simulink model "mux"  (R2023b)
settings: Solver=VariableStepAuto  StartTime=0.0  StopTime=1  RelTol=1e-3
settings Model: Creator=1234  LastModifiedBy=1234

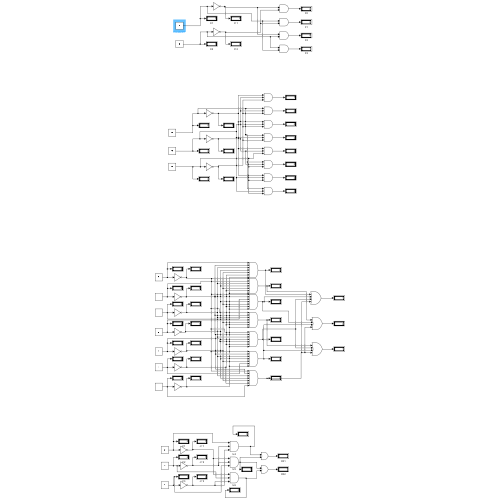
[thumbnail: Simulink's stored preview of the top-level diagram]
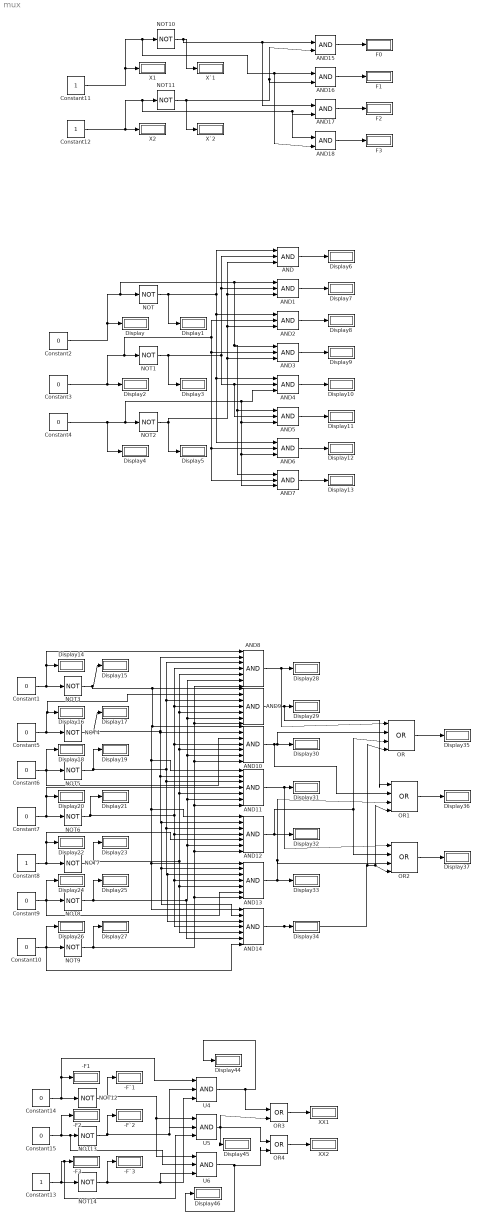
== system mux ==
  -F1 : Display
  -F2 : Display
  -F3 : Display
  -F`1 : Display
  -F`2 : Display
  -F`3 : Display
  AND{,1..7} (8 alike) : Logic  Inputs=3  IconShape=distinctive  AllPortsSameDT=off  OutDataTypeStr=boolean
  AND{8..14} (7 alike) : Logic  Inputs=7  IconShape=distinctive  AllPortsSameDT=off  OutDataTypeStr=boolean
  AND{15..18} (4 alike) : Logic  IconShape=distinctive  AllPortsSameDT=off  OutDataTypeStr=boolean
  Constant{1..7,9..10,14..15} (11 alike) : Constant  Value=0
  Constant{8,11..13} (4 alike) : Constant
  Display{,1..37,44..46} (41 alike) : Display
  F{0..3} (4 alike) : Display
  NOT{,1..14} (15 alike) : Logic  Operator=NOT  IconShape=distinctive  AllPortsSameDT=off  OutDataTypeStr=boolean
  OR : Logic  Operator=OR  Inputs=4  IconShape=distinctive  AllPortsSameDT=off  OutDataTypeStr=boolean
  OR1 : Logic  Operator=OR  Inputs=4  IconShape=distinctive  AllPortsSameDT=off  OutDataTypeStr=boolean
  OR2 : Logic  Operator=OR  Inputs=4  IconShape=distinctive  AllPortsSameDT=off  OutDataTypeStr=boolean
  OR3 : Logic  Operator=OR  IconShape=distinctive  AllPortsSameDT=off  OutDataTypeStr=boolean
  OR4 : Logic  Operator=OR  IconShape=distinctive  AllPortsSameDT=off  OutDataTypeStr=boolean
  U4 : Logic  Inputs=3  IconShape=distinctive  AllPortsSameDT=off  OutDataTypeStr=boolean
  U5 : Logic  Inputs=3  IconShape=distinctive  AllPortsSameDT=off  OutDataTypeStr=boolean
  U6 : Logic  Inputs=3  IconShape=distinctive  AllPortsSameDT=off  OutDataTypeStr=boolean
  X1 : Display
  X2 : Display
  XX1 : Display
  XX2 : Display
  X`1 : Display
  X`2 : Display
  wires:
  Constant2/1 -> AND7/1, AND5/1, AND3/1, AND1/1, NOT/1, Display/1
  NOT/1 -> AND/1, AND6/1, AND4/1, AND2/1, Display1/1
  NOT1/1 -> AND5/2, AND4/2, AND1/2, AND/2, Display3/1
  Constant3/1 -> AND2/2, AND6/2, AND7/2, AND3/2, NOT1/1, Display2/1
  NOT2/1 -> AND3/3, AND2/3, AND1/3, AND/3, Display5/1
  Constant4/1 -> Display4/1, AND5/3, AND6/3, AND7/3, AND4/3, NOT2/1
  AND/1 -> Display6/1
  AND2/1 -> Display8/1
  AND1/1 -> Display7/1
  AND3/1 -> Display9/1
  AND4/1 -> Display10/1
  AND5/1 -> Display11/1
  AND6/1 -> Display12/1
  AND7/1 -> Display13/1
  Constant1/1 -> AND8/1, Display14/1, NOT3/1
  Constant5/1 -> NOT4/1, AND9/2, Display16/1
  NOT6/1 -> AND14/4, AND13/4, AND12/4, AND10/4, AND9/4, AND8/4, Display21/1
  Constant7/1 -> AND11/4, Display20/1, NOT6/1
  Constant6/1 -> Display18/1, AND10/3, NOT5/1
  NOT8/1 -> AND14/6, AND12/6, AND11/6, AND10/6, AND9/6, AND8/6, Display25/1
  Constant9/1 -> AND13/6, Display24/1, NOT8/1
  Constant10/1 -> AND14/7, NOT9/1, Display26/1
  NOT9/1 -> AND13/7, AND12/7, AND11/7, AND10/7, AND9/7, AND8/7, Display27/1
  NOT7/1 -> AND11/5, AND10/5, AND9/5, AND8/5, AND14/5, AND13/5, Display23/1
  Constant8/1 -> AND12/5, Display22/1, NOT7/1
  NOT5/1 -> AND9/3, AND8/3, AND14/3, AND13/3, AND12/3, AND11/3, Display19/1
  NOT3/1 -> AND14/1, AND13/1, AND12/1, AND11/1, AND10/1, AND9/1, Display15/1
  NOT4/1 -> AND13/2, AND14/2, AND12/2, AND11/2, AND10/2, AND8/2, Display17/1
  AND8/1 -> OR/1, Display28/1
  AND9/1 -> OR1/1, Display29/1
  AND10/1 -> OR1/2, OR/2, Display30/1
  AND11/1 -> OR2/1, Display31/1
  AND12/1 -> OR2/2, OR/3, Display32/1
  AND13/1 -> OR1/3, OR2/3, Display33/1
  AND14/1 -> OR1/4, OR2/4, OR/4, Display34/1
  OR/1 -> Display35/1
  OR1/1 -> Display36/1
  OR2/1 -> Display37/1
  Constant12/1 -> X2/1, AND18/1, AND17/2, NOT11/1
  NOT11/1 -> AND16/2, AND15/2, X`2/1
  NOT10/1 -> AND17/1, AND15/1, X`1/1
  Constant11/1 -> X1/1, AND18/2, AND16/1, NOT10/1
  AND18/1 -> F3/1
  AND16/1 -> F1/1
  AND17/1 -> F2/1
  AND15/1 -> F0/1
  NOT12/1 -> U6/1, U5/1, -F`1/1
  NOT14/1 -> U6/3, U4/3, -F`3/1
  Constant15/1 -> U6/2, NOT13/1, -F2/1
  NOT13/1 -> U5/2, U4/2, -F`2/1
  Constant14/1 -> NOT12/1, U4/1, -F1/1
  Constant13/1 -> U5/3, -F3/1, NOT14/1
  U4/1 -> OR3/1, Display44/1
  U5/1 -> OR4/1, Display45/1, OR3/2
  U6/1 -> OR4/2, Display46/1
  OR3/1 -> XX1/1
  OR4/1 -> XX2/1
